simulink model "NPC_PV1"  (R2013a)
settings: Solver=FixedStepDiscrete  SolverMode=SingleTasking  StartTime=0.0  StopTime=Inf  FixedStep=Tpas  RelTol=1e-3
undefined symbols (not defined in the file): fmod4Q, IAFE3L, IDCP, Kac, Lac, PAFE3L, PDCP, Satv, Tpas, Vac
libraries: powerlib x40, simulink x12, powerlib_meascontrol x2
settings Model: Creator=LiberT  LastModifiedBy=Daniel
settings DataIOCC: SignalLoggingSaveFormat=ModelDataLogs
settings OptimizationCC: ExpressionDepthLimit=2147483647
settings DebuggingCC: MultiTaskDSMMsg=warning  MultiTaskCondExecSysMsg=none  FcnCallInpInsideContextMsg=EnableAllAsWarning  StrictBusMsg=None
settings RTWCC: IncludeERTFirstTime=on

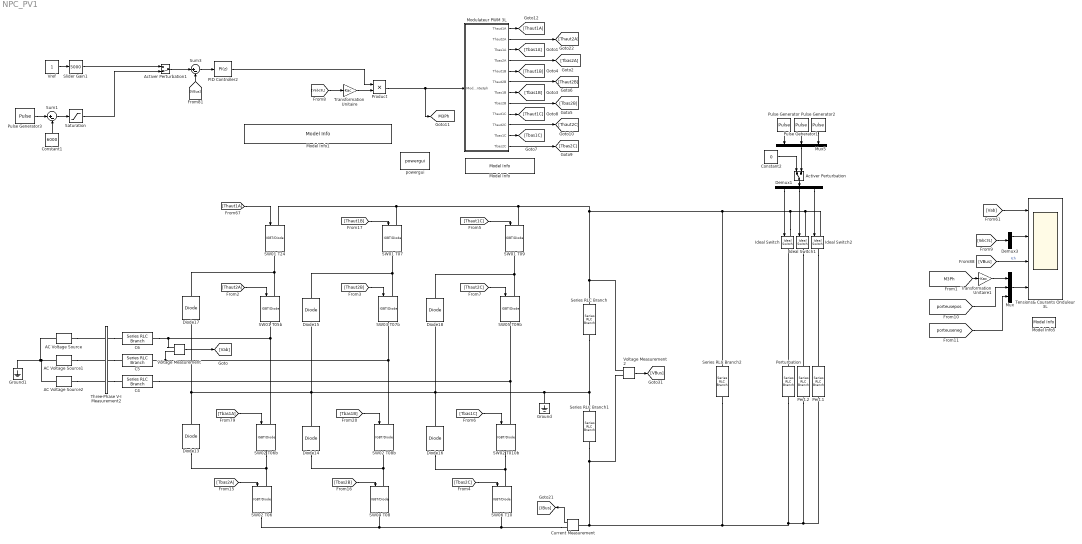
== system NPC_PV1 ==
  AC Voltage Source : powerlib/Electrical Sources/AC Voltage Source  Amplitude=Vac*sqrt(2/3)  Phase=0  Frequency=50  SampleTime=Tpas  Measurements=Voltage
  AC Voltage Source1 : powerlib/Electrical Sources/AC Voltage Source  Amplitude=Vac*sqrt(2/3)  Phase=-120  Frequency=50  SampleTime=Tpas  Measurements=Voltage
  AC Voltage Source2 : powerlib/Electrical Sources/AC Voltage Source  Amplitude=Vac*sqrt(2/3)  Phase=120  Frequency=50  SampleTime=Tpas  Measurements=Voltage
  Activer Perturbation : ManualSwitch
  Activer Perturbation1 : ManualSwitch  CurrentSetting=0
  C4 : powerlib/Elements/Series RLC Branch  LConnTagsString=__new0  RConnTagsString=__new0  BranchType=L  Resistance=10  Inductance=Lac  SetiL0=off  InitialCurrent=0  Capacitance=300e-3  Setx0=off  InitialVoltage=0  Measurements=None
  C5 : powerlib/Elements/Series RLC Branch  LConnTagsString=__new0  RConnTagsString=__new0  BranchType=L  Resistance=10  Inductance=Lac  SetiL0=off  InitialCurrent=0  Capacitance=300e-3  Setx0=off  InitialVoltage=0  Measurements=None
  C6 : powerlib/Elements/Series RLC Branch  LConnTagsString=__new0  RConnTagsString=__new0  BranchType=L  Resistance=10  Inductance=Lac  SetiL0=off  InitialCurrent=0  Capacitance=300e-3  Setx0=off  InitialVoltage=0  Measurements=None
  Constant1 : Constant  Value=6000
  Constant2 : Constant  Value=0
  Current Measurement : powerlib/Measurements/Current Measurement  PhasorSimulation=off  OutputType=Complex  PSBequivalent=0
  Demux1 : Demux  Outputs=3
  Demux3 : Demux  Outputs=3
  Diode{13..18} (6 alike) : powerlib/Power Electronics/Diode  Ron=0.001  Lon=0  Vf=0.8  IC=0  UseSnubber=off  Rs=500  Cs=inf  Measurements=off
  Ground : powerlib/Elements/Ground  LConnTagsString=a
  Ground1 : powerlib/Elements/Ground  LConnTagsString=a
  Ideal Switch : powerlib/Power Electronics/Ideal Switch  Ron=0.001  Lon=0  IC=0  Rs=1e5  Cs=inf  Measurements=off
  Ideal Switch1 : powerlib/Power Electronics/Ideal Switch  Ron=0.001  Lon=0  IC=0  Rs=1e5  Cs=inf  Measurements=off
  Ideal Switch2 : powerlib/Power Electronics/Ideal Switch  Ron=0.001  Lon=0  IC=0  Rs=1e5  Cs=inf  Measurements=off
  Model Info : simulink/Model-Wide Utilities/Model Info  InitialBlockCM=None  BlockCM=None  Frame=on  DisplayStringWithTags=Commande onduleur NPC3L  HorizontalTextAlignment=Center  LeftAlignmentValue=0.5  SourceBlockDiagram=NPC_PV1  TagMaxNumber=20
  Model Info1 : simulink/Model-Wide Utilities/Model Info  InitialBlockCM=None  BlockCM=None  Frame=off  DisplayStringWithTags=Générateur de modulantes triphasées d'amplitude variable  HorizontalTextAlignment=Center  LeftAlignmentValue=0.5  SourceBlockDiagram=NPC_PV1  TagMaxNumber=20
  Model Info5 : simulink/Model-Wide Utilities/Model Info  InitialBlockCM=None  BlockCM=None  Frame=on  DisplayStringWithTags=Résultats  HorizontalTextAlignment=Center  LeftAlignmentValue=0.5  SourceBlockDiagram=NPC_PV1  TagMaxNumber=20
  Modulateur PWM 3L : Subsystem
  Mux : Mux  Inputs=3
  Mux5 : Mux  Inputs=3
  PID Controller2 : simulink/Continuous/PID Controller  Controller=PI  TimeDomain=Discrete-time  SampleTime=Tpas  IntegratorMethod=Forward Euler  FilterMethod=Forward Euler  Form=Parallel  P=PAFE3L  I=IAFE3L  D=0  N=100  InitialConditionSource=internal  InitialConditionForIntegrator=0  InitialConditionForFilter=0  ExternalReset=none  LimitOutput=on  UpperSaturationLimit=Satv  LowerSaturationLimit=-Satv  LinearizeAsGain=on  AntiWindupMode=clamping  Kb=1  TrackingMode=off  Kt=1  PParamMin=[]  PParamMax=[]  IParamMin=[]  IParamMax=[]  DParamMin=[]  DParamMax=[]  NParamMin=[]  NParamMax=[]  KbParamMin=[]  KbParamMax=[]  KtParamMin=[]  KtParamMax=[]  POutMin=[]  POutMax=[]  IOutMin=[]  IOutMax=[]  DOutMin=[]  DOutMax=[]  NOutMin=[]  NOutMax=[]  KbOutMin=[]  KbOutMax=[]  KtOutMin=[]  KtOutMax=[]  IntegratorOutMin=[]  IntegratorOutMax=[]  FilterOutMin=[]  FilterOutMax=[]  SumOutMin=[]  SumOutMax=[]  SumI1OutMin=[]  SumI1OutMax=[]  SumI2OutMin=[]  SumI2OutMax=[]  SumI3OutMin=[]  SumI3OutMax=[]  SumDOutMin=[]  SumDOutMax=[]  SaturationOutMin=[]  SaturationOutMax=[]  IntegratorContinuousStateAttributes=''  IntegratorStateMustResolveToSignalObject=off  IntegratorRTWStateStorageClass=Auto  FilterContinuousStateAttributes=''  FilterStateMustResolveToSignalObject=off  FilterRTWStateStorageClass=Auto
  Pert.1 : powerlib/Elements/Series RLC Branch  LConnTagsString=__new0  RConnTagsString=__new0  BranchType=R  Resistance=20  Inductance=0  SetiL0=off  InitialCurrent=0  Capacitance=inf  Setx0=off  InitialVoltage=0  Measurements=None
  Pert.2 : powerlib/Elements/Series RLC Branch  LConnTagsString=__new0  RConnTagsString=__new0  BranchType=R  Resistance=20  Inductance=0  SetiL0=off  InitialCurrent=0  Capacitance=inf  Setx0=off  InitialVoltage=0  Measurements=None
  Perturbation : powerlib/Elements/Series RLC Branch  LConnTagsString=__new0  RConnTagsString=__new0  BranchType=R  Resistance=20  Inductance=0  SetiL0=off  InitialCurrent=0  Capacitance=inf  Setx0=off  InitialVoltage=0  Measurements=None
  Product : Product
  Pulse Generator : DiscretePulseGenerator  Period=floor((1/Tpas)/2)  PulseWidth=floor((1/Tpas)/4)  SampleTime=Tpas
  Pulse Generator1 : DiscretePulseGenerator  Period=floor((1/Tpas)/3)  PulseWidth=floor((1/Tpas)/6)  SampleTime=Tpas
  Pulse Generator2 : DiscretePulseGenerator  Period=floor((1/Tpas))  PulseWidth=floor((1/Tpas)/2)  SampleTime=Tpas
  Pulse Generator3 : DiscretePulseGenerator  Amplitude=12000  Period=floor(.4/Tpas)  PulseWidth=floor(.4/2/Tpas)  SampleTime=Tpas
  SW01 T05b : powerlib/Power Electronics/IGBT//Diode  Ron=1e-3  Rs=1e5  Cs=Tpas  Measurements=off
  SW01 T07 : powerlib/Power Electronics/IGBT//Diode  Ron=1e-3  Rs=1e5  Cs=Tpas  Measurements=off
  SW01 T09 : powerlib/Power Electronics/IGBT//Diode  Ron=1e-3  Rs=1e5  Cs=Tpas  Measurements=off
  SW01 T24 : powerlib/Power Electronics/IGBT//Diode  Ron=1e-3  Rs=1e5  Cs=Tpas  Measurements=off
  SW02 T010b : powerlib/Power Electronics/IGBT//Diode  Ron=1e-3  Rs=1e5  Cs=Tpas  Measurements=off
  SW02 T06 : powerlib/Power Electronics/IGBT//Diode  Ron=1e-3  Rs=1e5  Cs=Tpas  Measurements=off
  SW02 T06b : powerlib/Power Electronics/IGBT//Diode  Ron=1e-3  Rs=1e5  Cs=Tpas  Measurements=off
  SW02 T08b : powerlib/Power Electronics/IGBT//Diode  Ron=1e-3  Rs=1e5  Cs=Tpas  Measurements=off
  SW03 T07b : powerlib/Power Electronics/IGBT//Diode  Ron=1e-3  Rs=1e5  Cs=Tpas  Measurements=off
  SW04 T08 : powerlib/Power Electronics/IGBT//Diode  Ron=1e-3  Rs=1e5  Cs=Tpas  Measurements=off
  SW05 T09b : powerlib/Power Electronics/IGBT//Diode  Ron=1e-3  Rs=1e5  Cs=Tpas  Measurements=off
  SW06 T10 : powerlib/Power Electronics/IGBT//Diode  Ron=1e-3  Rs=1e5  Cs=Tpas  Measurements=off
  Saturation : Saturate  UpperLimit=5100  LowerLimit=5000
  Series RLC Branch : powerlib/Elements/Series RLC Branch  LConnTagsString=__new0  RConnTagsString=__new0  BranchType=C  Resistance=1  Inductance=1e-3  SetiL0=off  InitialCurrent=0  Capacitance=660e-3  Setx0=on  InitialVoltage=2500  Measurements=None
  Series RLC Branch1 : powerlib/Elements/Series RLC Branch  LConnTagsString=__new0  RConnTagsString=__new0  BranchType=C  Resistance=1  Inductance=1e-3  SetiL0=off  InitialCurrent=0  Capacitance=660e-3  Setx0=on  InitialVoltage=2500  Measurements=None
  Series RLC Branch2 : powerlib/Elements/Series RLC Branch  LConnTagsString=__new0  RConnTagsString=__new0  BranchType=R  Resistance=9.26  Inductance=1e-3  SetiL0=off  InitialCurrent=0  Capacitance=660e-3  Setx0=on  InitialVoltage=2500  Measurements=None
  Slider Gain1 : simulink/Math Operations/Slider Gain  low=0  gain=5000  high=7000
  Sum1 : Sum  Inputs=|+-
  Sum3 : Sum  Inputs=|+-
  Tensions& Courants Onduleur 3L : Scope  NumInputPorts=4
      settings: TickLabels=on  ShowLegends=on  TimeRange=1  YMin=-7500~-3000~4990~-1  YMax=7500~3000~5110~1  SaveName=ScopeData2
  Three-Phase V-I Measurement2 : powerlib/Measurements/Three-Phase V-I Measurement  VoltageMeasurement=phase-to-ground  SetLabelV=on  LabelV=Vabc3L  Vpu=off  VpuLL=off  CurrentMeasurement=yes  SetLabelI=on  LabelI=Iabc3L  Ipu=off  Pbase=100e6  Vbase=500e3  OutputType=Complex  PhasorSimulation=off  PSBequivalent=0
  Transformation Unitaire : Gain  Gain=-Kac
  Transformation Unitaire1 : Gain  Gain=-Kac
  Voltage Measurement : powerlib/Measurements/Voltage Measurement  PhasorSimulation=off  OutputType=Complex  PSBequivalent=0
  Voltage Measurement2 : powerlib/Measurements/Voltage Measurement  PhasorSimulation=off  OutputType=Complex  PSBequivalent=0
  Vref : Constant  SampleTime=Tpas
  powergui : powerlib/powergui  Priority=1  SimulationMode=Discrete  SolverType=Tustin  SampleTime=Tpas  frequency=60  SPID=off  DisableSnubberDevices=off  DisableRonSwitches=off  DisableVfSwitches=off  SwTol=0  Interpol=off  DisplayEquations=off  frequencyindice=0  Pbase=100e6  ErrMax=1e-4  Iterations=50  UnitsV=kV  UnitsW=MW  FunctionMessages=off  echomessages=off  HookPort=off  EnableUseOfTLC=off  x0status=blocks  RestoreLinks=warning  ResistiveCurrentMeasurement=off  Frange=[0:2:500]  Ylog=off  Xlog=on  ShowGrid=off  save=off  variable=ZData  structure=ScopeData1  ZoomFFT=off  StartTime=18  cycles=100  DisplayStyle=1  fundamental=50  FreqAxis=off  MaxFrequency=2000  frequencyindicesteady=1  RmsSteady=1  display=off  Ts=0  methode=off
  tag scope: M3Ph=global
  wires:
  Current Measurement/1 -> [IBus]
  [Thaut1A] -> SW01 T24/1
  [Tbas1A] -> SW02 T06b/1
  [Tbas2A] -> SW02 T06/1
  [Thaut1B] -> SW01 T07/1
  [Tbas1B] -> SW02 T08b/1
  [Tbas2B] -> SW04 T08/1
  Product/1 -> [M3Ph], Modulateur PWM 3L/1(Modulante3ph)
  Voltage Measurement2/1 -> [VBus]
  Modulateur PWM 3L/1(Thaut1A) -> [Thaut1A]
  Modulateur PWM 3L/2(Thaut2A) -> [Thaut2A]
  Modulateur PWM 3L/3(Tbas1A) -> [Tbas1A]
  Modulateur PWM 3L/4(Tbas2A) -> [Tbas2A]
  Modulateur PWM 3L/5(Thaut1B) -> [Thaut1B]
  Modulateur PWM 3L/6(Thaut2B) -> [Thaut2B]
  Modulateur PWM 3L/7(Tbas1B) -> [Tbas1B]
  Modulateur PWM 3L/8(Tbas2B) -> [Tbas2B]
  Modulateur PWM 3L/9(Thaut1C) -> [Thaut1C]
  Modulateur PWM 3L/10(Thaut2C) -> [Thaut2C]
  Modulateur PWM 3L/11(Tbas1C) -> [Tbas1C]
  [Thaut2A] -> SW01 T05b/1
  [Thaut2B] -> SW03 T07b/1
  [Thaut1C] -> SW01 T09/1
  [Thaut2C] -> SW05 T09b/1
  [Tbas1C] -> SW02 T010b/1
  [Tbas2C] -> SW06 T10/1
  [Vabc3L] -> Transformation Unitaire/1
  Transformation Unitaire/1 -> Product/2
  Modulateur PWM 3L/12(Tbas2C) -> [Tbas2C]
  [VBus] -> Tensions& Courants Onduleur 3L/3  "Ich"
  [Iabc3L] -> Demux3/1
  Demux3/1 -> Tensions& Courants Onduleur 3L/2
  Mux/1 -> Tensions& Courants Onduleur 3L/4
  [porteusepos] -> Mux/2
  [porteuseneg] -> Mux/3
  [VBus] -> Sum3/2
  Vref/1 -> Slider Gain1/1
  Sum3/1 -> PID Controller2/1
  PID Controller2/1 -> Product/1
  Voltage Measurement/1 -> [Vab]
  [Vab] -> Tensions& Courants Onduleur 3L/1
  [M3Ph] -> Transformation Unitaire1/1
  Transformation Unitaire1/1 -> Mux/1
  Demux1/1 -> Ideal Switch/1
  Demux1/2 -> Ideal Switch1/1
  Demux1/3 -> Ideal Switch2/1
  Pulse Generator/1 -> Mux5/1
  Pulse Generator1/1 -> Mux5/2
  Pulse Generator2/1 -> Mux5/3
  Activer Perturbation/1 -> Demux1/1
  Mux5/1 -> Activer Perturbation/2
  Constant2/1 -> Activer Perturbation/1
  Sum1/1 -> Saturation/1
  Pulse Generator3/1 -> Sum1/1
  Constant1/1 -> Sum1/2
  Activer Perturbation1/1 -> Sum3/1
  Slider Gain1/1 -> Activer Perturbation1/1
  Saturation/1 -> Activer Perturbation1/2
  connections:
  Perturbation/RConn1 -- Current Measurement/LConn1 -- Series RLC Branch1/RConn1 -- Voltage Measurement2/LConn2 -- Series RLC Branch2/RConn1 -- Pert.1/RConn1 -- Pert.2/RConn1
  Ideal Switch/LConn1 -- Series RLC Branch2/LConn1 -- SW01 T07/LConn1 -- SW01 T24/LConn1 -- SW01 T09/LConn1 -- Series RLC Branch/LConn1 -- Voltage Measurement2/LConn1 -- Ideal Switch1/LConn1 -- Ideal Switch2/LConn1
  Ground/LConn1 -- Diode16/RConn1 -- Diode18/LConn1 -- Diode15/LConn1 -- Diode14/RConn1 -- Diode13/RConn1 -- Diode17/LConn1 -- Series RLC Branch1/LConn1 -- Series RLC Branch/RConn1
  SW02 T06b/LConn1 -- C6/LConn1 -- Voltage Measurement/LConn1 -- SW01 T05b/RConn1
  SW02 T010b/LConn1 -- C4/LConn1 -- SW05 T09b/RConn1
  SW03 T07b/RConn1 -- C5/LConn1 -- Voltage Measurement/LConn2 -- SW02 T08b/LConn1
  Diode17/RConn1 -- SW01 T24/RConn1 -- SW01 T05b/LConn1
  Diode15/RConn1 -- SW01 T07/RConn1 -- SW03 T07b/LConn1
  Diode18/RConn1 -- SW01 T09/RConn1 -- SW05 T09b/LConn1
  Diode13/LConn1 -- SW02 T06/LConn1 -- SW02 T06b/RConn1
  Diode16/LConn1 -- SW06 T10/LConn1 -- SW02 T010b/RConn1
  Diode14/LConn1 -- SW02 T08b/RConn1 -- SW04 T08/LConn1
  Current Measurement/RConn1 -- SW06 T10/RConn1 -- SW04 T08/RConn1 -- SW02 T06/RConn1
  AC Voltage Source/LConn1 -- AC Voltage Source2/LConn1 -- AC Voltage Source1/LConn1 -- Ground1/LConn1
  AC Voltage Source/RConn1 -- Three-Phase V-I Measurement2/RConn1
  AC Voltage Source1/RConn1 -- Three-Phase V-I Measurement2/RConn2
  AC Voltage Source2/RConn1 -- Three-Phase V-I Measurement2/RConn3
  Three-Phase V-I Measurement2/LConn1 -- C6/RConn1
  Three-Phase V-I Measurement2/LConn2 -- C5/RConn1
  Three-Phase V-I Measurement2/LConn3 -- C4/RConn1
  Ideal Switch1/RConn1 -- Pert.2/LConn1
  Ideal Switch2/RConn1 -- Pert.1/LConn1
  Perturbation/LConn1 -- Ideal Switch/RConn1

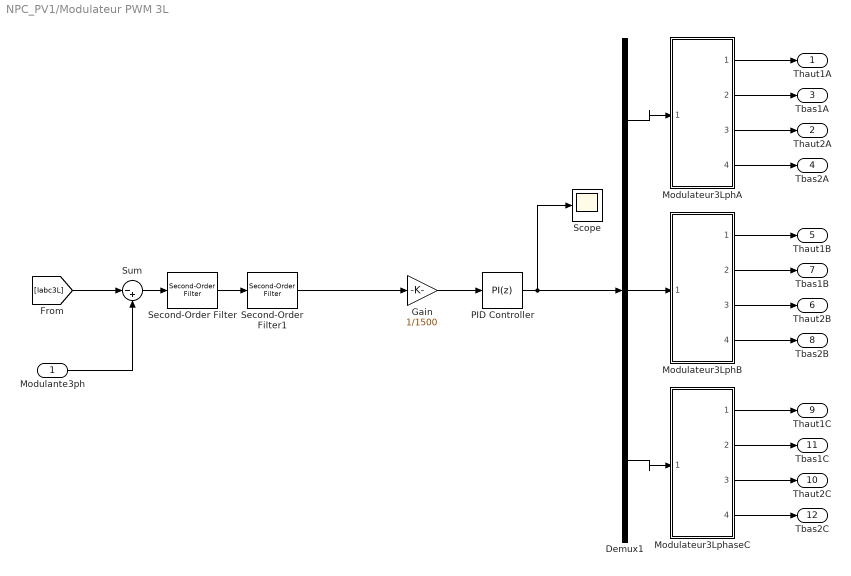
== system NPC_PV1/Modulateur PWM 3L ==
  Modulante3ph : Inport
  Demux1 : Demux  Outputs=3
  Gain : Gain  Gain=1/1500
  "Modulateur3LphA " : Subsystem
  Modulateur3LphB : Subsystem
  Modulateur3LphaseC : Subsystem
  PID Controller : simulink/Continuous/PID Controller  Controller=PI  TimeDomain=Discrete-time  SampleTime=Tpas  IntegratorMethod=Forward Euler  FilterMethod=Forward Euler  Form=Parallel  P=PDCP  I=IDCP  D=0  N=100  InitialConditionSource=internal  InitialConditionForIntegrator=0  InitialConditionForFilter=0  ExternalReset=none  LimitOutput=on  UpperSaturationLimit=0.98  LowerSaturationLimit=-0.98  LinearizeAsGain=on  AntiWindupMode=none  Kb=1  TrackingMode=off  Kt=1  PParamMin=[]  PParamMax=[]  IParamMin=[]  IParamMax=[]  DParamMin=[]  DParamMax=[]  NParamMin=[]  NParamMax=[]  KbParamMin=[]  KbParamMax=[]  KtParamMin=[]  KtParamMax=[]  POutMin=[]  POutMax=[]  IOutMin=[]  IOutMax=[]  DOutMin=[]  DOutMax=[]  NOutMin=[]  NOutMax=[]  KbOutMin=[]  KbOutMax=[]  KtOutMin=[]  KtOutMax=[]  IntegratorOutMin=[]  IntegratorOutMax=[]  FilterOutMin=[]  FilterOutMax=[]  SumOutMin=[]  SumOutMax=[]  SumI1OutMin=[]  SumI1OutMax=[]  SumI2OutMin=[]  SumI2OutMax=[]  SumI3OutMin=[]  SumI3OutMax=[]  SumDOutMin=[]  SumDOutMax=[]  SaturationOutMin=[]  SaturationOutMax=[]  IntegratorContinuousStateAttributes=''  IntegratorStateMustResolveToSignalObject=off  IntegratorRTWStateStorageClass=Auto  FilterContinuousStateAttributes=''  FilterStateMustResolveToSignalObject=off  FilterRTWStateStorageClass=Auto
  Scope : Scope
      settings: TimeRange=0.02  YMin=-0.9  YMax=0.9
  Second-Order Filter : powerlib_meascontrol/Filters/Second-Order Filter  FilterType=Lowpass  Fo=1e3*1.25  Zeta=1  Ts=Tpas  Initialize=on  Vac_Init="[0,  0,  50]"  Vdc_Init=0  PlotResponse=off  FreqRange=[0, 10000, 1]
  Second-Order Filter1 : powerlib_meascontrol/Filters/Second-Order Filter  FilterType=Lowpass  Fo=1e3*1.25  Zeta=1  Ts=Tpas  Initialize=on  Vac_Init="[0,  0,  50]"  Vdc_Init=0  PlotResponse=off  FreqRange=[0, 10000, 1]
  Sum : Sum  Inputs=|-+
  Thaut1A : Outport
  Thaut2A : Outport  Port=2
  Tbas1A : Outport  Port=3
  Tbas2A : Outport  Port=4
  Thaut1B : Outport  Port=5
  Thaut2B : Outport  Port=6
  Tbas1B : Outport  Port=7
  Tbas2B : Outport  Port=8
  Thaut1C : Outport  Port=9
  Thaut2C : Outport  Port=10
  Tbas1C : Outport  Port=11
  Tbas2C : Outport  Port=12
  wires:
  Demux1/1 -> "Modulateur3LphA "/1(Modulante)
  "Modulateur3LphA "/1(Thaut1) -> Thaut1A/1
  "Modulateur3LphA "/2(Tbas1) -> Tbas1A/1
  "Modulateur3LphA "/3(Thaut2) -> Thaut2A/1
  "Modulateur3LphA "/4(Tbas2) -> Tbas2A/1
  Demux1/2 -> Modulateur3LphB/1(Modulante)
  Modulateur3LphB/1(Thaut1) -> Thaut1B/1
  Modulateur3LphB/2(Tbas1) -> Tbas1B/1
  Modulateur3LphB/3(Thaut2) -> Thaut2B/1
  Modulateur3LphB/4(Tbas2) -> Tbas2B/1
  Demux1/3 -> Modulateur3LphaseC/1(Modulante)
  Modulateur3LphaseC/1(Thaut1) -> Thaut1C/1
  Modulateur3LphaseC/2(Tbas1) -> Tbas1C/1
  Modulateur3LphaseC/3(Thaut2) -> Thaut2C/1
  Modulateur3LphaseC/4(Tbas2) -> Tbas2C/1
  Modulante3ph/1 -> Sum/2
  PID Controller/1 -> Scope/1, Demux1/1
  Sum/1 -> Second-Order Filter/1
  Second-Order Filter/1 -> Second-Order Filter1/1
  [Iabc3L] -> Sum/1
  Gain/1 -> PID Controller/1
  Second-Order Filter1/1 -> Gain/1

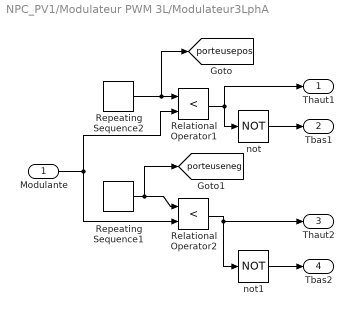
== system NPC_PV1/Modulateur PWM 3L/Modulateur3LphA  ==
  Modulante : Inport
  Relational Operator1 : RelationalOperator  Operator=<  OutDataTypeStr=boolean
  Relational Operator2 : RelationalOperator  Operator=<  OutDataTypeStr=boolean
  Repeating Sequence1 : simulink/Sources/Repeating Sequence  rep_seq_t=[0 .5/fmod4Q 1/fmod4Q]  rep_seq_y=[-1 0 -1]
  Repeating Sequence2 : simulink/Sources/Repeating Sequence  rep_seq_t=[0 .5/fmod4Q 1/fmod4Q]  rep_seq_y=[0 1 0]
  not : Logic  Operator=NOT  IconShape=distinctive  AllPortsSameDT=off  OutDataTypeStr=boolean
  not1 : Logic  Operator=NOT  IconShape=distinctive  AllPortsSameDT=off  OutDataTypeStr=boolean
  Thaut1 : Outport
  Tbas1 : Outport  Port=2
  Thaut2 : Outport  Port=3
  Tbas2 : Outport  Port=4
  tag scope: porteuseneg=global, porteusepos=global
  wires:
  Repeating Sequence2/1 -> [porteusepos], Relational Operator1/1
  Modulante/1 -> Relational Operator1/2, Relational Operator2/2
  Repeating Sequence1/1 -> [porteuseneg], Relational Operator2/1
  Relational Operator1/1 -> not/1, Thaut1/1
  not/1 -> Tbas1/1
  not1/1 -> Tbas2/1
  Relational Operator2/1 -> not1/1, Thaut2/1

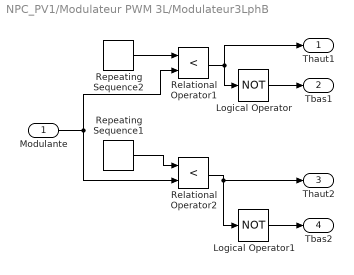
== system NPC_PV1/Modulateur PWM 3L/Modulateur3LphB ==
  Modulante : Inport
  Logical Operator : Logic  Operator=NOT  AllPortsSameDT=off  OutDataTypeStr=boolean
  Logical Operator1 : Logic  Operator=NOT  AllPortsSameDT=off  OutDataTypeStr=boolean
  Relational Operator1 : RelationalOperator  Operator=<  OutDataTypeStr=boolean
  Relational Operator2 : RelationalOperator  Operator=<  OutDataTypeStr=boolean
  Repeating Sequence1 : simulink/Sources/Repeating Sequence  rep_seq_t=[0 .5/fmod4Q 1/fmod4Q]  rep_seq_y=[-1 0 -1]
  Repeating Sequence2 : simulink/Sources/Repeating Sequence  rep_seq_t=[0 .5/fmod4Q 1/fmod4Q]  rep_seq_y=[0 1 0]
  Thaut1 : Outport
  Tbas1 : Outport  Port=2
  Thaut2 : Outport  Port=3
  Tbas2 : Outport  Port=4
  wires:
  Repeating Sequence2/1 -> Relational Operator1/1
  Modulante/1 -> Relational Operator1/2, Relational Operator2/2
  Repeating Sequence1/1 -> Relational Operator2/1
  Relational Operator1/1 -> Logical Operator/1, Thaut1/1
  Logical Operator/1 -> Tbas1/1
  Logical Operator1/1 -> Tbas2/1
  Relational Operator2/1 -> Logical Operator1/1, Thaut2/1

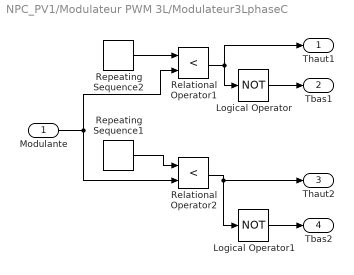
== system NPC_PV1/Modulateur PWM 3L/Modulateur3LphaseC ==
  Modulante : Inport
  Logical Operator : Logic  Operator=NOT  AllPortsSameDT=off  OutDataTypeStr=boolean
  Logical Operator1 : Logic  Operator=NOT  AllPortsSameDT=off  OutDataTypeStr=boolean
  Relational Operator1 : RelationalOperator  Operator=<  OutDataTypeStr=boolean
  Relational Operator2 : RelationalOperator  Operator=<  OutDataTypeStr=boolean
  Repeating Sequence1 : simulink/Sources/Repeating Sequence  rep_seq_t=[0 .5/fmod4Q 1/fmod4Q]  rep_seq_y=[-1 0 -1]
  Repeating Sequence2 : simulink/Sources/Repeating Sequence  rep_seq_t=[0 .5/fmod4Q 1/fmod4Q]  rep_seq_y=[0 1 0]
  Thaut1 : Outport
  Tbas1 : Outport  Port=2
  Thaut2 : Outport  Port=3
  Tbas2 : Outport  Port=4
  wires:
  Repeating Sequence2/1 -> Relational Operator1/1
  Modulante/1 -> Relational Operator1/2, Relational Operator2/2
  Repeating Sequence1/1 -> Relational Operator2/1
  Relational Operator1/1 -> Logical Operator/1, Thaut1/1
  Logical Operator/1 -> Tbas1/1
  Logical Operator1/1 -> Tbas2/1
  Relational Operator2/1 -> Logical Operator1/1, Thaut2/1
